simulink model "Energization"  (R2020a)
settings: Solver=VariableStepAuto  StartTime=0.0  StopTime=0.3  RelTol=1e-3
libraries: powerlib x18
settings Model: Creator=Alisamar  LastModifiedBy=Alisamar

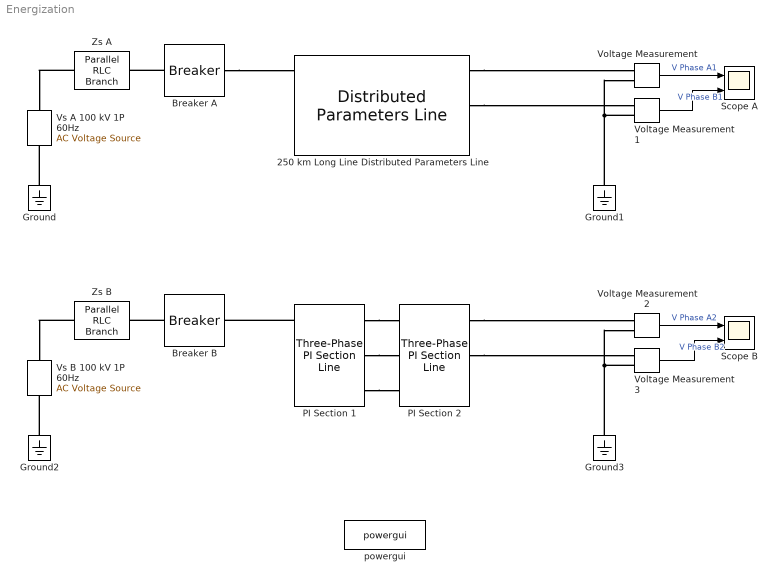
== system Energization ==
  250 km Long Line Distributed Parameters Line : powerlib/Elements/Distributed Parameters Line  Phases=3  Frequency=60  Resistance=[0.01273 0.3864]  Inductance="[0.9337e-3  4.1264e-3]"  Capacitance=[12.74e-9 7.751e-9]  Length=250  x1=[0 0 0;376.991118430775 376.991118430775 376.991118430775;0 0 0]  x2=[0 0 0;376.991118430775 376.991118430775 376.991118430775;0 0 0]  x3=[0 0 0;376.991118430775 376.991118430775 376.991118430775;0 0 0]  x4=[0 0 0;376.991118430775 376.991118430775 376.991118430775;0 0 0]  x5=0.00141385391748936  V1=[0 0 0;377 377 377;0 0 0]  V2=[0 0 0;377 377 377;0 0 0]  I1=[0 0 0;377 377 377;0 0 0]  I2=[0 0 0;377 377 377;0 0 0]  nHarmo=1  Measurements=None
  Breaker A : powerlib/Elements/Breaker  InitialState=0  SwitchingTimes="[5/60  10/60]"  External=off  BreakerResistance=0.01  SnubberResistance=1e6  SnubberCapacitance=0  Measurements=None  MoreParameters=on  NoBreakLoop=off
  Breaker B : powerlib/Elements/Breaker  InitialState=0  SwitchingTimes=[5/60 10/60]  External=off  BreakerResistance=0.01  SnubberResistance=1e6  SnubberCapacitance=0  Measurements=None  MoreParameters=on  NoBreakLoop=off
  Ground{,1..3} (4 alike) : powerlib/Elements/Ground  LConnTagsString=a
  PI Section 1 : powerlib/Elements/Three-Phase PI Section Line  LConnTagsString=a|b|c  RConnTagsString=A|B|C  Frequency=60  Resistances=[ 0.01273 0.3864]  Inductances="[ 0.9337e-3  4.1264e-3]"  Capacitances=[12.74e-9 7.751e-9]  Length=125
  PI Section 2 : powerlib/Elements/Three-Phase PI Section Line  LConnTagsString=a|b|c  RConnTagsString=A|B|C  Frequency=60  Resistances=[ 0.01273 0.3864]  Inductances="[ 0.9337e-3  4.1264e-3]"  Capacitances=[12.74e-9 7.751e-9]  Length=125
  Scope A : Scope  NumInputPorts=2
  Scope B : Scope  NumInputPorts=2
  Voltage Measurement{,1..3} (4 alike) : powerlib/Measurements/Voltage Measurement  PhasorSimulation=off  OutputType=Complex  PSBequivalent=0
  Vs A 100 kV 1P 60Hz : powerlib/Electrical Sources/AC Voltage Source  Amplitude=100e3  Phase=0  Frequency=60  SampleTime=0  Measurements=None  BusType=swing  Pref=10e3  Qref=0  Qmin=-inf  Qmax=+inf
  Vs B 100 kV 1P 60Hz : powerlib/Electrical Sources/AC Voltage Source  Amplitude=100e3  Phase=0  Frequency=60  SampleTime=0  Measurements=None  BusType=swing  Pref=10e3  Qref=0  Qmin=-inf  Qmax=+inf
  Zs A : powerlib/Elements/Parallel RLC Branch  LConnTagsString=a  RConnTagsString=__new0  BranchType=RL  Resistance=1  Inductance=1e-3  SetiL0=off  InitialCurrent=0  Capacitance=1e-6  Setx0=off  InitialVoltage=0  Measurements=None
  Zs B : powerlib/Elements/Parallel RLC Branch  LConnTagsString=a  RConnTagsString=__new0  BranchType=RL  Resistance=1  Inductance=1e-3  SetiL0=off  InitialCurrent=0  Capacitance=1e-6  Setx0=off  InitialVoltage=0  Measurements=None
  powergui : powerlib/powergui  Priority=1  SimulationMode=Continuous  SampleTime=50e-6  frequency=60  Iterations=50  frequencyindice=60  Pbase=100e6  ErrMax=1e-4  UnitsV=kV  UnitsW=MW  buscounter=0  FunctionMessages=off  echomessages=off  EnableUseOfTLC=off  CurrentSourceSwitches=off  DisableSnubberDevices=off  DisableRonSwitches=off  DisableVfSwitches=off  DisplayEquations=off  AutomaticDiscreteSolvers=off  SolverType=Tustin/Backward Euler (TBE)  Interpol=off  ExternalGateDelay=off  methode=off  Ts=100  x0status=blocks  SPID=on  SwTol=0  HookPort=off  NonlinearTolerance=1e-4  nMaxIteration=100  ContinueOnMaxIteration=off  RestoreLinks=warning  ResistiveCurrentMeasurement=off  Frange=[0:2:500]  Ylog=off  Xlog=on  ShowGrid=off  save=off  variable=ZData  structure=0  ZoomFFT=off  StartTime=0.0  cycles=1  DisplayStyle=1  fundamental=60  FreqAxis=off  MaxFrequency=1000  frequencyindicesteady=1  RmsSteady=1  display=off
  wires:
  Voltage Measurement1/1 -> Scope A/2  "V Phase B1"
  Voltage Measurement/1 -> Scope A/1  "V Phase A1"
  Voltage Measurement2/1 -> Scope B/1  "V Phase A2"
  Voltage Measurement3/1 -> Scope B/2  "V Phase B2"
  connections:
  Breaker A/LConn1 -- Zs A/RConn1
  Breaker A/RConn1 -- 250 km Long Line Distributed Parameters Line/LConn1
  250 km Long Line Distributed Parameters Line/RConn1 -- Voltage Measurement/LConn1
  Zs A/LConn1 -- Vs A 100 kV 1P 60Hz/RConn1
  Ground1/LConn1 -- Voltage Measurement/LConn2 -- Voltage Measurement1/LConn2
  250 km Long Line Distributed Parameters Line/RConn2 -- Voltage Measurement1/LConn1
  Ground/LConn1 -- Vs A 100 kV 1P 60Hz/LConn1
  Voltage Measurement3/LConn2 -- Ground3/LConn1 -- Voltage Measurement2/LConn2
  Ground2/LConn1 -- Vs B 100 kV 1P 60Hz/LConn1
  PI Section 1/LConn1 -- Breaker B/RConn1
  Zs B/LConn1 -- Vs B 100 kV 1P 60Hz/RConn1
  Breaker B/LConn1 -- Zs B/RConn1
  PI Section 1/RConn1 -- PI Section 2/LConn1
  PI Section 1/RConn2 -- PI Section 2/LConn2
  PI Section 1/RConn3 -- PI Section 2/LConn3
  PI Section 2/RConn1 -- Voltage Measurement2/LConn1
  PI Section 2/RConn2 -- Voltage Measurement3/LConn1
